simulink model "TwoLegRobotSim"  (R2022b)
settings: Solver=VariableStepAuto  StartTime=0.0  StopTime=20  MaxStep=1e-4  MinStep=1e-6  RelTol=1e-3
model workspace: external: MATLAB File D:\5720\Tutorial 2\TwoLegRobot_DataFile.m (data not in the file)
undefined symbols (not defined in the file): base_params, current_params, k_cols, k_rows, Mass_body, Mass_lower_leg, Mass_upper_leg, Mass_wheel, P0, p_matrix, qphi, qth, qx, R_k, smiData, X, X0_hat, Y, Z
libraries: sm_lib x79, nesl_utility x17, slpidlib x5
(part 1 of 4)
settings Model: Creator=Lyn20  LastModifiedBy=Lyn20

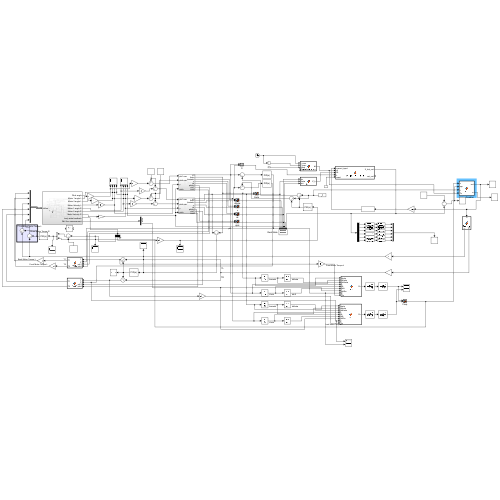
[thumbnail: Simulink's stored preview of the top-level diagram]
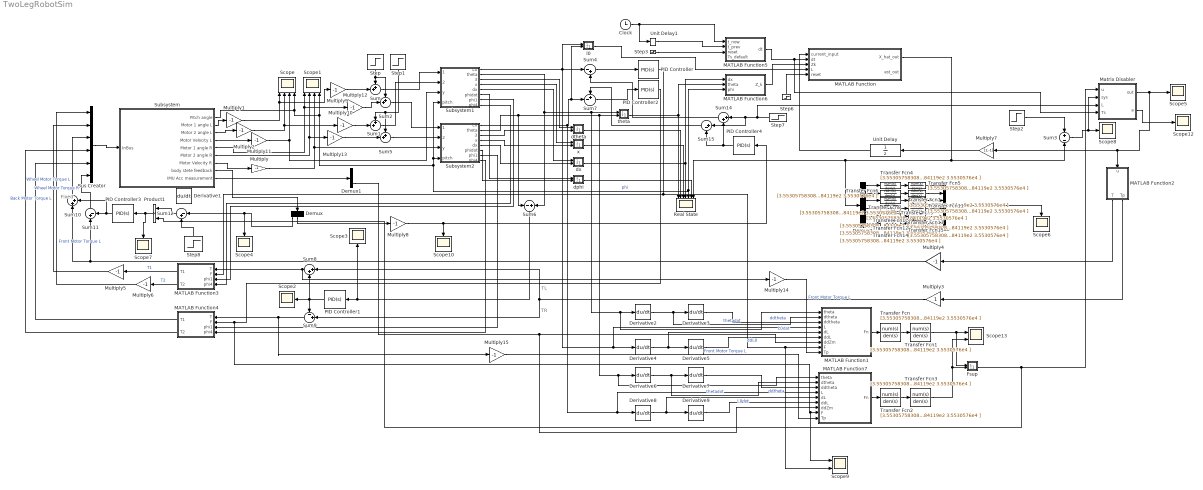
== system TwoLegRobotSim ==
  note: Fixed
  note: TR
  note: TL
  Bus Creator : BusCreator  Inputs=6
  Clock : Clock
  Demux : Demux  Outputs=3
  Demux1 : Demux  Outputs=3
  Demux2 : Demux  Outputs=6
  Derivative{1..9} (9 alike) : Derivative
  Fsup : MATLAB Function  TreatAsAtomicUnit=on
  MATLAB Function : MATLAB Function  TreatAsAtomicUnit=on
  MATLAB Function1 : MATLAB Function  TreatAsAtomicUnit=on
  MATLAB Function2 : MATLAB Function  TreatAsAtomicUnit=on
  MATLAB Function3 : MATLAB Function  TreatAsAtomicUnit=on
  MATLAB Function4 : MATLAB Function  TreatAsAtomicUnit=on
  MATLAB Function5 : MATLAB Function  TreatAsAtomicUnit=on
  MATLAB Function6 : MATLAB Function  TreatAsAtomicUnit=on
  MATLAB Function7 : MATLAB Function  TreatAsAtomicUnit=on
  Matrix Disabler : MATLAB Function  TreatAsAtomicUnit=on
  Multiply{,1..2,4..6,8..15} (14 alike) : Gain  Gain=-1
  Multiply3 : Gain
  Multiply7 : Gain  Gain=[1;-1]
  Mux : Mux  Inputs=6
  PID Controller : slpidlib/PID Controller  Controller=PID  Form=Parallel  TimeDomain=Continuous-time  UseExternalTs=off  SampleTime=0.01  IntegratorMethod=Forward Euler  FilterMethod=Forward Euler  ControllerParametersSource=internal  P=2000  I=-20  UseKiTs=off  D=100  N=100  UseFilter=on  TunerSelectOption=Transfer Function Based (PID Tuner App)  InitialConditionSource=internal  InitialConditionForIntegrator=0  InitialConditionForFilter=0  DifferentiatorICPrevScaledInput=0  ExternalReset=none  TrackingMode=off  Kt=1  LimitOutput=off  SatLimitsSource=internal  UpperSaturationLimit=inf  LowerSaturationLimit=-inf  LinearizeAsGain=on  AntiWindupMode=none  Kb=1  LimitIntegrator=off  UpperIntegratorSaturationLimit=inf  LowerIntegratorSaturationLimit=-inf  POutMin=[]  POutMax=[]  IOutMin=[]  IOutMax=[]  DOutMin=[]  DOutMax=[]  NOutMin=[]  NOutMax=[]  SumOutMin=[]  SumOutMax=[]  SaturationOutMin=[]  SaturationOutMax=[]  PParamMin=[]  PParamMax=[]  IParamMin=[]  IParamMax=[]  DParamMin=[]  DParamMax=[]  NParamMin=[]  NParamMax=[]  KbParamMin=[]  KbParamMax=[]  KtParamMin=[]  KtParamMax=[]  KbOutMin=[]  KbOutMax=[]  KtOutMin=[]  KtOutMax=[]  IntegratorOutMin=[]  IntegratorOutMax=[]  FilterOutMin=[]  FilterOutMax=[]  SumI1OutMin=[]  SumI1OutMax=[]  SumI2OutMin=[]  SumI2OutMax=[]  SumI3OutMin=[]  SumI3OutMax=[]  SumI4OutMin=[]  SumI4OutMax=[]  SumDOutMin=[]  SumDOutMax=[]  DifferentiatorOutMin=[]  DifferentiatorOutMax=[]  FilterDiffOutCoefMin=[]  FilterDiffOutCoefMax=[]  ReciprocalOutMin=[]  ReciprocalOutMax=[]  SumDenOutMin=[]  SumDenOutMax=[]  SumNumOutMin=[]  SumNumOutMax=[]  DivideOutMin=[]  DivideOutMax=[]  UdiffTsProdOutMin=[]  UdiffTsProdOutMax=[]  NTsProdOutMin=[]  NTsProdOutMax=[]  UintegralTsProdOutMin=[]  UintegralTsProdOutMax=[]  UngainTsProdOutMin=[]  UngainTsProdOutMax=[]  ClampingZeroOutDataTypeStr=Inherit: Inherit via back propagation  ClampingZeroOutMin=[]  ClampingZeroOutMax=[]  FilterDenConstantOutDataTypeStr=Inherit: Inherit via back propagation  FilterDenConstantOutMin=[]  FilterDenConstantOutMax=[]  PCopyOutDataTypeStr=Inherit: Inherit via back propagation  PCopyOutMin=[]  PCopyOutMax=[]  NCopyOutDataTypeStr=Inherit: Inherit via back propagation  NCopyOutMin=[]  NCopyOutMax=[]  IntegratorContinuousStateAttributes=''  IntegratorStateMustResolveToSignalObject=off  IntegratorRTWStateStorageClass=Auto  FilterContinuousStateAttributes=''  FilterStateMustResolveToSignalObject=off  FilterRTWStateStorageClass=Auto  ParallelPVariant=InternalParameters  IdealPVariant=Disabled  IVariant=InternalParameters  DVariant=InternalParameters  IntegratorVariant=Continuous  SatVariant=Disabled  AWVariant=Passthrough  PCopyVariant=Disabled  TRVariant=Disabled  FdbkBlocksVariant=Forward  IdealPFdbkVariant=Disabled  SatFdbkVariant=Disabled  DerivativeFilterVariant=ContFilter  NVariant=InternalParameters  NCopyVariant=Disabled  FilterICVariant=InternalICsFilter  IntegratorICVariant=InternalICs  ExternalResetVariant=Disabled  TRSumVariant=Passthrough  SumFdbkVariant=Disabled  SumVariant=Sum_PID  TsampFilterVariant=InternalTs  TsampNgainVariant=Passthrough  TsampIntegralVariant=Passthrough  ExternalSaturationOutDataTypeStr=Inherit: Same as second input
  PID Controller1 : slpidlib/PID Controller  Controller=PID  Form=Parallel  TimeDomain=Continuous-time  UseExternalTs=off  SampleTime=0.01  IntegratorMethod=Forward Euler  FilterMethod=Forward Euler  ControllerParametersSource=internal  P=30  I=0.5  UseKiTs=off  D=3  N=100  UseFilter=on  TunerSelectOption=Transfer Function Based (PID Tuner App)  InitialConditionSource=internal  InitialConditionForIntegrator=0  InitialConditionForFilter=0  DifferentiatorICPrevScaledInput=0  ExternalReset=none  TrackingMode=off  Kt=1  LimitOutput=off  SatLimitsSource=internal  UpperSaturationLimit=inf  LowerSaturationLimit=-inf  LinearizeAsGain=on  AntiWindupMode=none  Kb=1  LimitIntegrator=off  UpperIntegratorSaturationLimit=inf  LowerIntegratorSaturationLimit=-inf  POutMin=[]  POutMax=[]  IOutMin=[]  IOutMax=[]  DOutMin=[]  DOutMax=[]  NOutMin=[]  NOutMax=[]  SumOutMin=[]  SumOutMax=[]  SaturationOutMin=[]  SaturationOutMax=[]  PParamMin=[]  PParamMax=[]  IParamMin=[]  IParamMax=[]  DParamMin=[]  DParamMax=[]  NParamMin=[]  NParamMax=[]  KbParamMin=[]  KbParamMax=[]  KtParamMin=[]  KtParamMax=[]  KbOutMin=[]  KbOutMax=[]  KtOutMin=[]  KtOutMax=[]  IntegratorOutMin=[]  IntegratorOutMax=[]  FilterOutMin=[]  FilterOutMax=[]  SumI1OutMin=[]  SumI1OutMax=[]  SumI2OutMin=[]  SumI2OutMax=[]  SumI3OutMin=[]  SumI3OutMax=[]  SumI4OutMin=[]  SumI4OutMax=[]  SumDOutMin=[]  SumDOutMax=[]  DifferentiatorOutMin=[]  DifferentiatorOutMax=[]  FilterDiffOutCoefMin=[]  FilterDiffOutCoefMax=[]  ReciprocalOutMin=[]  ReciprocalOutMax=[]  SumDenOutMin=[]  SumDenOutMax=[]  SumNumOutMin=[]  SumNumOutMax=[]  DivideOutMin=[]  DivideOutMax=[]  UdiffTsProdOutMin=[]  UdiffTsProdOutMax=[]  NTsProdOutMin=[]  NTsProdOutMax=[]  UintegralTsProdOutMin=[]  UintegralTsProdOutMax=[]  UngainTsProdOutMin=[]  UngainTsProdOutMax=[]  ClampingZeroOutDataTypeStr=Inherit: Inherit via back propagation  ClampingZeroOutMin=[]  ClampingZeroOutMax=[]  FilterDenConstantOutDataTypeStr=Inherit: Inherit via back propagation  FilterDenConstantOutMin=[]  FilterDenConstantOutMax=[]  PCopyOutDataTypeStr=Inherit: Inherit via back propagation  PCopyOutMin=[]  PCopyOutMax=[]  NCopyOutDataTypeStr=Inherit: Inherit via back propagation  NCopyOutMin=[]  NCopyOutMax=[]  IntegratorContinuousStateAttributes=''  IntegratorStateMustResolveToSignalObject=off  IntegratorRTWStateStorageClass=Auto  FilterContinuousStateAttributes=''  FilterStateMustResolveToSignalObject=off  FilterRTWStateStorageClass=Auto  ParallelPVariant=InternalParameters  IdealPVariant=Disabled  IVariant=InternalParameters  DVariant=InternalParameters  IntegratorVariant=Continuous  SatVariant=Disabled  AWVariant=Passthrough  PCopyVariant=Disabled  TRVariant=Disabled  FdbkBlocksVariant=Forward  IdealPFdbkVariant=Disabled  SatFdbkVariant=Disabled  DerivativeFilterVariant=ContFilter  NVariant=InternalParameters  NCopyVariant=Disabled  FilterICVariant=InternalICsFilter  IntegratorICVariant=InternalICs  ExternalResetVariant=Disabled  TRSumVariant=Passthrough  SumFdbkVariant=Disabled  SumVariant=Sum_PID  TsampFilterVariant=InternalTs  TsampNgainVariant=Passthrough  TsampIntegralVariant=Passthrough  ExternalSaturationOutDataTypeStr=Inherit: Same as second input
  PID Controller2 : slpidlib/PID Controller  Controller=PID  Form=Parallel  TimeDomain=Continuous-time  UseExternalTs=off  SampleTime=0.01  IntegratorMethod=Forward Euler  FilterMethod=Forward Euler  ControllerParametersSource=internal  P=2000  I=-20  UseKiTs=off  D=100  N=100  UseFilter=on  TunerSelectOption=Transfer Function Based (PID Tuner App)  InitialConditionSource=internal  InitialConditionForIntegrator=0  InitialConditionForFilter=0  DifferentiatorICPrevScaledInput=0  ExternalReset=none  TrackingMode=off  Kt=1  LimitOutput=off  SatLimitsSource=internal  UpperSaturationLimit=inf  LowerSaturationLimit=-inf  LinearizeAsGain=on  AntiWindupMode=none  Kb=1  LimitIntegrator=off  UpperIntegratorSaturationLimit=inf  LowerIntegratorSaturationLimit=-inf  POutMin=[]  POutMax=[]  IOutMin=[]  IOutMax=[]  DOutMin=[]  DOutMax=[]  NOutMin=[]  NOutMax=[]  SumOutMin=[]  SumOutMax=[]  SaturationOutMin=[]  SaturationOutMax=[]  PParamMin=[]  PParamMax=[]  IParamMin=[]  IParamMax=[]  DParamMin=[]  DParamMax=[]  NParamMin=[]  NParamMax=[]  KbParamMin=[]  KbParamMax=[]  KtParamMin=[]  KtParamMax=[]  KbOutMin=[]  KbOutMax=[]  KtOutMin=[]  KtOutMax=[]  IntegratorOutMin=[]  IntegratorOutMax=[]  FilterOutMin=[]  FilterOutMax=[]  SumI1OutMin=[]  SumI1OutMax=[]  SumI2OutMin=[]  SumI2OutMax=[]  SumI3OutMin=[]  SumI3OutMax=[]  SumI4OutMin=[]  SumI4OutMax=[]  SumDOutMin=[]  SumDOutMax=[]  DifferentiatorOutMin=[]  DifferentiatorOutMax=[]  FilterDiffOutCoefMin=[]  FilterDiffOutCoefMax=[]  ReciprocalOutMin=[]  ReciprocalOutMax=[]  SumDenOutMin=[]  SumDenOutMax=[]  SumNumOutMin=[]  SumNumOutMax=[]  DivideOutMin=[]  DivideOutMax=[]  UdiffTsProdOutMin=[]  UdiffTsProdOutMax=[]  NTsProdOutMin=[]  NTsProdOutMax=[]  UintegralTsProdOutMin=[]  UintegralTsProdOutMax=[]  UngainTsProdOutMin=[]  UngainTsProdOutMax=[]  ClampingZeroOutDataTypeStr=Inherit: Inherit via back propagation  ClampingZeroOutMin=[]  ClampingZeroOutMax=[]  FilterDenConstantOutDataTypeStr=Inherit: Inherit via back propagation  FilterDenConstantOutMin=[]  FilterDenConstantOutMax=[]  PCopyOutDataTypeStr=Inherit: Inherit via back propagation  PCopyOutMin=[]  PCopyOutMax=[]  NCopyOutDataTypeStr=Inherit: Inherit via back propagation  NCopyOutMin=[]  NCopyOutMax=[]  IntegratorContinuousStateAttributes=''  IntegratorStateMustResolveToSignalObject=off  IntegratorRTWStateStorageClass=Auto  FilterContinuousStateAttributes=''  FilterStateMustResolveToSignalObject=off  FilterRTWStateStorageClass=Auto  ParallelPVariant=InternalParameters  IdealPVariant=Disabled  IVariant=InternalParameters  DVariant=InternalParameters  IntegratorVariant=Continuous  SatVariant=Disabled  AWVariant=Passthrough  PCopyVariant=Disabled  TRVariant=Disabled  FdbkBlocksVariant=Forward  IdealPFdbkVariant=Disabled  SatFdbkVariant=Disabled  DerivativeFilterVariant=ContFilter  NVariant=InternalParameters  NCopyVariant=Disabled  FilterICVariant=InternalICsFilter  IntegratorICVariant=InternalICs  ExternalResetVariant=Disabled  TRSumVariant=Passthrough  SumFdbkVariant=Disabled  SumVariant=Sum_PID  TsampFilterVariant=InternalTs  TsampNgainVariant=Passthrough  TsampIntegralVariant=Passthrough  ExternalSaturationOutDataTypeStr=Inherit: Same as second input
  PID Controller3 : slpidlib/PID Controller  Controller=PID  Form=Parallel  TimeDomain=Continuous-time  UseExternalTs=off  SampleTime=0.01  IntegratorMethod=Forward Euler  FilterMethod=Forward Euler  ControllerParametersSource=internal  P=10  I=1  UseKiTs=off  D=1  N=100  UseFilter=on  TunerSelectOption=Transfer Function Based (PID Tuner App)  InitialConditionSource=internal  InitialConditionForIntegrator=0  InitialConditionForFilter=0  DifferentiatorICPrevScaledInput=0  ExternalReset=none  TrackingMode=off  Kt=1  LimitOutput=off  SatLimitsSource=internal  UpperSaturationLimit=inf  LowerSaturationLimit=-inf  LinearizeAsGain=on  AntiWindupMode=none  Kb=1  LimitIntegrator=off  UpperIntegratorSaturationLimit=inf  LowerIntegratorSaturationLimit=-inf  POutMin=[]  POutMax=[]  IOutMin=[]  IOutMax=[]  DOutMin=[]  DOutMax=[]  NOutMin=[]  NOutMax=[]  SumOutMin=[]  SumOutMax=[]  SaturationOutMin=[]  SaturationOutMax=[]  PParamMin=[]  PParamMax=[]  IParamMin=[]  IParamMax=[]  DParamMin=[]  DParamMax=[]  NParamMin=[]  NParamMax=[]  KbParamMin=[]  KbParamMax=[]  KtParamMin=[]  KtParamMax=[]  KbOutMin=[]  KbOutMax=[]  KtOutMin=[]  KtOutMax=[]  IntegratorOutMin=[]  IntegratorOutMax=[]  FilterOutMin=[]  FilterOutMax=[]  SumI1OutMin=[]  SumI1OutMax=[]  SumI2OutMin=[]  SumI2OutMax=[]  SumI3OutMin=[]  SumI3OutMax=[]  SumI4OutMin=[]  SumI4OutMax=[]  SumDOutMin=[]  SumDOutMax=[]  DifferentiatorOutMin=[]  DifferentiatorOutMax=[]  FilterDiffOutCoefMin=[]  FilterDiffOutCoefMax=[]  ReciprocalOutMin=[]  ReciprocalOutMax=[]  SumDenOutMin=[]  SumDenOutMax=[]  SumNumOutMin=[]  SumNumOutMax=[]  DivideOutMin=[]  DivideOutMax=[]  UdiffTsProdOutMin=[]  UdiffTsProdOutMax=[]  NTsProdOutMin=[]  NTsProdOutMax=[]  UintegralTsProdOutMin=[]  UintegralTsProdOutMax=[]  UngainTsProdOutMin=[]  UngainTsProdOutMax=[]  ClampingZeroOutDataTypeStr=Inherit: Inherit via back propagation  ClampingZeroOutMin=[]  ClampingZeroOutMax=[]  FilterDenConstantOutDataTypeStr=Inherit: Inherit via back propagation  FilterDenConstantOutMin=[]  FilterDenConstantOutMax=[]  PCopyOutDataTypeStr=Inherit: Inherit via back propagation  PCopyOutMin=[]  PCopyOutMax=[]  NCopyOutDataTypeStr=Inherit: Inherit via back propagation  NCopyOutMin=[]  NCopyOutMax=[]  IntegratorContinuousStateAttributes=''  IntegratorStateMustResolveToSignalObject=off  IntegratorRTWStateStorageClass=Auto  FilterContinuousStateAttributes=''  FilterStateMustResolveToSignalObject=off  FilterRTWStateStorageClass=Auto  ParallelPVariant=InternalParameters  IdealPVariant=Disabled  IVariant=InternalParameters  DVariant=InternalParameters  IntegratorVariant=Continuous  SatVariant=Disabled  AWVariant=Passthrough  PCopyVariant=Disabled  TRVariant=Disabled  FdbkBlocksVariant=Forward  IdealPFdbkVariant=Disabled  SatFdbkVariant=Disabled  DerivativeFilterVariant=ContFilter  NVariant=InternalParameters  NCopyVariant=Disabled  FilterICVariant=InternalICsFilter  IntegratorICVariant=InternalICs  ExternalResetVariant=Disabled  TRSumVariant=Passthrough  SumFdbkVariant=Disabled  SumVariant=Sum_PID  TsampFilterVariant=InternalTs  TsampNgainVariant=Passthrough  TsampIntegralVariant=Passthrough  ExternalSaturationOutDataTypeStr=Inherit: Same as second input
  PID Controller4 : slpidlib/PID Controller  Controller=PID  Form=Parallel  TimeDomain=Continuous-time  UseExternalTs=off  SampleTime=-1  IntegratorMethod=Forward Euler  FilterMethod=Forward Euler  ControllerParametersSource=internal  P=20  I=1  UseKiTs=off  D=0  N=100  UseFilter=on  TunerSelectOption=Transfer Function Based (PID Tuner App)  InitialConditionSource=internal  InitialConditionForIntegrator=0  InitialConditionForFilter=0  DifferentiatorICPrevScaledInput=0  ExternalReset=none  TrackingMode=off  Kt=1  LimitOutput=off  SatLimitsSource=internal  UpperSaturationLimit=inf  LowerSaturationLimit=-inf  LinearizeAsGain=on  AntiWindupMode=none  Kb=1  LimitIntegrator=off  UpperIntegratorSaturationLimit=inf  LowerIntegratorSaturationLimit=-inf  POutMin=[]  POutMax=[]  IOutMin=[]  IOutMax=[]  DOutMin=[]  DOutMax=[]  NOutMin=[]  NOutMax=[]  SumOutMin=[]  SumOutMax=[]  SaturationOutMin=[]  SaturationOutMax=[]  PParamMin=[]  PParamMax=[]  IParamMin=[]  IParamMax=[]  DParamMin=[]  DParamMax=[]  NParamMin=[]  NParamMax=[]  KbParamMin=[]  KbParamMax=[]  KtParamMin=[]  KtParamMax=[]  KbOutMin=[]  KbOutMax=[]  KtOutMin=[]  KtOutMax=[]  IntegratorOutMin=[]  IntegratorOutMax=[]  FilterOutMin=[]  FilterOutMax=[]  SumI1OutMin=[]  SumI1OutMax=[]  SumI2OutMin=[]  SumI2OutMax=[]  SumI3OutMin=[]  SumI3OutMax=[]  SumI4OutMin=[]  SumI4OutMax=[]  SumDOutMin=[]  SumDOutMax=[]  DifferentiatorOutMin=[]  DifferentiatorOutMax=[]  FilterDiffOutCoefMin=[]  FilterDiffOutCoefMax=[]  ReciprocalOutMin=[]  ReciprocalOutMax=[]  SumDenOutMin=[]  SumDenOutMax=[]  SumNumOutMin=[]  SumNumOutMax=[]  DivideOutMin=[]  DivideOutMax=[]  UdiffTsProdOutMin=[]  UdiffTsProdOutMax=[]  NTsProdOutMin=[]  NTsProdOutMax=[]  UintegralTsProdOutMin=[]  UintegralTsProdOutMax=[]  UngainTsProdOutMin=[]  UngainTsProdOutMax=[]  ClampingZeroOutDataTypeStr=Inherit: Inherit via back propagation  ClampingZeroOutMin=[]  ClampingZeroOutMax=[]  FilterDenConstantOutDataTypeStr=Inherit: Inherit via back propagation  FilterDenConstantOutMin=[]  FilterDenConstantOutMax=[]  PCopyOutDataTypeStr=Inherit: Inherit via back propagation  PCopyOutMin=[]  PCopyOutMax=[]  NCopyOutDataTypeStr=Inherit: Inherit via back propagation  NCopyOutMin=[]  NCopyOutMax=[]  IntegratorContinuousStateAttributes=''  IntegratorStateMustResolveToSignalObject=off  IntegratorRTWStateStorageClass=Auto  FilterContinuousStateAttributes=''  FilterStateMustResolveToSignalObject=off  FilterRTWStateStorageClass=Auto  ParallelPVariant=InternalParameters  IdealPVariant=Disabled  IVariant=InternalParameters  DVariant=InternalParameters  IntegratorVariant=Continuous  SatVariant=Disabled  AWVariant=Passthrough  PCopyVariant=Disabled  TRVariant=Disabled  FdbkBlocksVariant=Forward  IdealPFdbkVariant=Disabled  SatFdbkVariant=Disabled  DerivativeFilterVariant=ContFilter  NVariant=InternalParameters  NCopyVariant=Disabled  FilterICVariant=InternalICsFilter  IntegratorICVariant=InternalICs  ExternalResetVariant=Disabled  TRSumVariant=Passthrough  SumFdbkVariant=Disabled  SumVariant=Sum_PID  TsampFilterVariant=InternalTs  TsampNgainVariant=Passthrough  TsampIntegralVariant=Passthrough  ExternalSaturationOutDataTypeStr=Inherit: Same as second input
  Product1 : Product
  Real State : Scope  NumInputPorts=7
  Scope : Scope  NumInputPorts=4
  Scope1 : Scope  NumInputPorts=4
  Scope{2..8,10,12} (9 alike) : Scope
  Scope13 : Scope  NumInputPorts=2
  Scope9 : Scope  NumInputPorts=2
  Step : Step  Time=0  After=1.5*pi  SampleTime=0
  Step1 : Step  Time=0  After=0.5*pi  SampleTime=0
  Step2 : Step  Time=20  Before=[0;0.35;0;0;0;0]  After=[0;-0.35;0;0;0;0]  SampleTime=0
  Step3 : Step  Time=0  After=0  SampleTime=0
  Step6 : Step  Time=0  After=0  SampleTime=0
  Step7 : Step  Time=10  Before=0.23  After=0.23  SampleTime=0
  Step8 : Step  Time=0.75  After=0  SampleTime=0
  Subsystem : Subsystem
  Subsystem1 : Subsystem
  Subsystem2 : Subsystem
  Sum{,1..2,5} (4 alike) : Sum  Inputs=++|
  Sum10 : Sum  Inputs=|++
  Sum11 : Sum  Inputs=|+-
  Sum12 : Sum  Inputs=|-+
  Sum14 : Sum  Inputs=|++
  Sum15 : Sum  Inputs=|+-
  Sum3 : Sum  Inputs=+|-
  Sum4 : Sum  Inputs=|-+
  Sum6 : Sum  Inputs=-|+
  Sum7 : Sum  Inputs=+-|
  Sum8 : Sum  Inputs=|++
  Sum9 : Sum  Inputs=-+|
  Transfer Fcn{,1..15} (16 alike) : TransferFcn  Numerator=[3.553057583087056e4]  Denominator=[ 1 3.484119e2 3.5530576e4 ]
  Unit Delay : UnitDelay  SampleTime=-1  HasFrameUpgradeWarning=on
  Unit Delay1 : UnitDelay  SampleTime=1e-4  HasFrameUpgradeWarning=on
  dphi : MATLAB Function  TreatAsAtomicUnit=on
  dtheta : MATLAB Function  TreatAsAtomicUnit=on
  dx : MATLAB Function  TreatAsAtomicUnit=on
  l0 : MATLAB Function  TreatAsAtomicUnit=on
  theta : MATLAB Function  TreatAsAtomicUnit=on
  x : MATLAB Function  TreatAsAtomicUnit=on
  wires:
  Subsystem/2(Motor 1 angle L) -> Multiply1/1
  Subsystem/3(Motor 2 angle L) -> Multiply2/1
  Subsystem/4(Motor Velocity L) -> Multiply11/1
  Subsystem1/1(L0) -> MATLAB Function1/4(L), Derivative4/1, Sum4/1, l0/1(u1)
  dphi/1(y) -> Real State/6
  x/1(y) -> Real State/3
  MATLAB Function2/2(Tp) -> Multiply3/1
  Multiply3/1 -> Sum8/1, Sum9/2
  theta/1(y) -> Real State/1, MATLAB Function6/2(theta)
  dx/1(y) -> Real State/4, MATLAB Function6/1(dx)
  MATLAB Function2/1(T) -> Multiply4/1
  Subsystem/1(Pitch angle) -> Scope1/4, Subsystem1/4(pitch), Subsystem2/4(pitch), MATLAB Function6/3(phi), Real State/5, Scope/4  "phi"
  Sum3/1 -> Scope8/1, Matrix Disabler/2(sys)
  Sum4/1 -> PID Controller/1
  Step2/1 -> Sum3/1
  PID Controller/1 -> MATLAB Function3/2(F), Scope9/2, MATLAB Function1/8(F)
  dtheta/1(y) -> Real State/2
  MATLAB Function3/2(T2) -> Multiply6/1  "T2"
  MATLAB Function3/1(T1) -> Multiply5/1  "T1"
  Subsystem/6(Motor 2 angle R) -> Scope1/2, Multiply13/1
  Subsystem/7(Motor Velocity R) -> Multiply/1
  Subsystem/5(Motor 1 angle R) -> Scope1/1, Multiply12/1
  Multiply/1 -> Subsystem2/3(y), Scope1/3
  Multiply1/1 -> Scope/1, Multiply9/1
  Multiply2/1 -> Scope/2, Multiply10/1
  Multiply9/1 -> Sum/2
  Sum/1 -> Subsystem1/1(phi1 raw)
  Multiply10/1 -> Sum1/2
  Sum1/1 -> Subsystem1/2(phi4 raw)
  Step/1 -> Sum2/1, Sum/1
  Step1/1 -> Sum5/1, Sum1/1
  Multiply4/1 -> Sum11/1, Sum10/1
  Multiply11/1 -> Subsystem1/3(y), Scope/3
  Multiply12/1 -> Sum2/2
  Sum2/1 -> Subsystem2/1(phi1 raw)
  Multiply13/1 -> Sum5/2
  Sum5/1 -> Subsystem2/2(phi4 raw)
  Subsystem1/2(theta) -> Sum6/2, MATLAB Function1/1(theta), Derivative2/1, theta/1(u1)
  Subsystem1/3(thetadot) -> dtheta/1(u1)
  Subsystem1/4(x) -> x/1(u1)
  Subsystem1/5(dx) -> dx/1(u1)
  Subsystem1/6(phidot) -> dphi/1(u1)
  Subsystem1/8(phi4) -> MATLAB Function3/4(phi4)
  Subsystem2/1(L0) -> MATLAB Function7/4(L), Derivative8/1, l0/2(u2), Sum7/2
  Subsystem2/2(theta) -> Sum6/1, MATLAB Function7/1(theta), Derivative6/1, theta/2(u2)
  Subsystem2/3(thetadot) -> dtheta/2(u2)
  Subsystem2/4(x) -> x/2(u2)
  Subsystem2/5(dx) -> dx/2(u2)
  Subsystem2/6(phidot) -> dphi/2(u2)
  Subsystem2/8(phi4) -> MATLAB Function4/4(phi4)
  Sum6/1 -> PID Controller1/1, Scope3/1
  Subsystem1/7(phi1) -> MATLAB Function3/3(phi1)
  Subsystem2/7(phi1) -> MATLAB Function4/3(phi1)
  Sum7/1 -> PID Controller2/1
  PID Controller2/1 -> Scope9/1, MATLAB Function7/8(F), MATLAB Function4/2(F)
  Sum8/1 -> MATLAB Function3/1(T), Multiply14/1
  PID Controller1/1 -> Sum9/1, Scope2/1, Sum8/2
  Sum9/1 -> Multiply15/1, MATLAB Function4/1(T)
  Subsystem/8(body stete feedback) -> Demux/1
  Sum12/1 -> Product1/1
  Demux/1 -> Sum12/1, Scope4/1
  Step8/1 -> Sum12/2
  Clock/1 -> Unit Delay1/1, MATLAB Function5/1(t_now)
  MATLAB Function5/1(dt) -> Matrix Disabler/4(Ts), MATLAB Function/2(dt)
  Step3/1 -> MATLAB Function5/3(reset)
  MATLAB Function6/1(Z_k) -> MATLAB Function/3(Zk)
  Step6/1 -> MATLAB Function/5(reset)
  Unit Delay/1 -> MATLAB Function/1(current_input)
  Unit Delay1/1 -> MATLAB Function5/2(t_prev)
  Multiply6/1 -> Bus Creator/1  "Front Motor Torque L"
  Multiply5/1 -> Bus Creator/2  "Back Motor Torque L"
  Sum10/1 -> Bus Creator/3  "Wheel Motor Torque L"
  MATLAB Function4/2(T2) -> Bus Creator/4
  MATLAB Function4/1(T1) -> Bus Creator/5
  Sum11/1 -> Bus Creator/6  "Wheel Motor Torque R"
  Bus Creator/1 -> Subsystem/1(InBus)
  Matrix Disabler/1(out) -> Multiply7/1, MATLAB Function2/1(u), Scope5/1
  l0/1(y) -> MATLAB Function/4(L)
  Multiply7/1 -> Unit Delay/1
  Step7/1 -> Sum15/1, Sum14/1, Matrix Disabler/3(L)
  Demux/2 -> Multiply8/1
  Multiply8/1 -> PID Controller4/1, Scope10/1
  Sum14/1 -> Sum4/2
  Sum15/1 -> Sum7/1
  PID Controller4/1 -> Sum15/2, Sum14/2
  Matrix Disabler/2(a) -> Scope12/1
  Subsystem/9(IMU Acc measurement) -> Demux1/1
  Derivative2/1 -> MATLAB Function1/2(dtheta), Derivative3/1  "thetadot"
  Derivative4/1 -> MATLAB Function1/5(dL), Derivative5/1  "L0dot"
  Derivative3/1 -> MATLAB Function1/3(ddtheta)  "ddtheta"
  Derivative7/1 -> MATLAB Function7/3(ddtheta)  "ddtheta"
  Derivative9/1 -> MATLAB Function7/6(ddL)
  Derivative8/1 -> MATLAB Function7/5(dL), Derivative9/1  "L0dot"
  Derivative6/1 -> MATLAB Function7/2(dtheta), Derivative7/1  "thetadot"
  Derivative5/1 -> MATLAB Function1/6(ddL)  "ddL0"
  Demux1/3 -> MATLAB Function1/7(ddZm), MATLAB Function7/7(ddZm)
  Transfer Fcn/1 -> Transfer Fcn1/1
  MATLAB Function1/1(Fn) -> Transfer Fcn/1
  Transfer Fcn1/1 -> Fsup/1(u1), Scope13/1
  Transfer Fcn3/1 -> Fsup/2(u2), Scope13/2
  Transfer Fcn2/1 -> Transfer Fcn3/1
  MATLAB Function7/1(Fn) -> Transfer Fcn2/1
  Multiply14/1 -> MATLAB Function1/9(Tp)  "Front Motor Torque L"
  Multiply15/1 -> MATLAB Function7/9(Tp)  "Front Motor Torque L"
  Fsup/1(y) -> Product1/2, Matrix Disabler/1(u)
  Transfer Fcn4/1 -> Transfer Fcn5/1
  MATLAB Function/1(X_hat_out) -> Demux2/1, Real State/7, Sum3/2
  Transfer Fcn5/1 -> Mux/1
  Demux2/1 -> Transfer Fcn4/1
  Transfer Fcn6/1 -> Transfer Fcn7/1
  Demux2/2 -> Transfer Fcn6/1
  Transfer Fcn7/1 -> Mux/2
  Transfer Fcn8/1 -> Transfer Fcn9/1
  Demux2/3 -> Transfer Fcn8/1
  Transfer Fcn9/1 -> Mux/3
  Transfer Fcn10/1 -> Transfer Fcn11/1
  Transfer Fcn15/1 -> Mux/6
  Demux2/4 -> Transfer Fcn10/1
  Demux2/6 -> Transfer Fcn14/1
  Transfer Fcn14/1 -> Transfer Fcn15/1
  Transfer Fcn12/1 -> Transfer Fcn13/1
  Demux2/5 -> Transfer Fcn12/1
  Transfer Fcn13/1 -> Mux/5
  Transfer Fcn11/1 -> Mux/4
  Mux/1 -> Scope6/1
  PID Controller3/1 -> Sum10/2, Sum11/2
  Product1/1 -> Scope7/1, PID Controller3/1
